simulink model "EPD_China_3_gen_without_limits"  (R2021b)
settings: Solver=VariableStepAuto  StartTime=0.0  StopTime=2  RelTol=1e-3
settings Model: Creator=vijay  LastModifiedBy=vijay

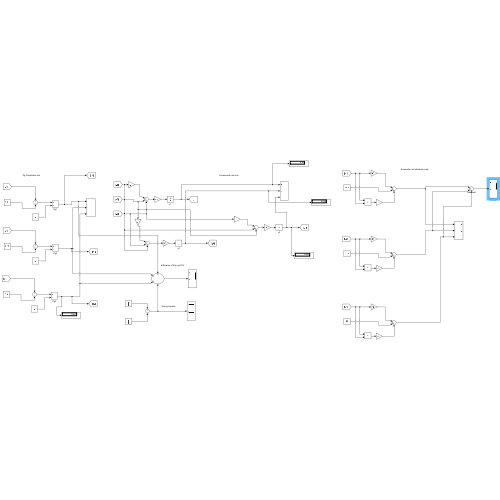
[thumbnail: Simulink's stored preview of the top-level diagram]
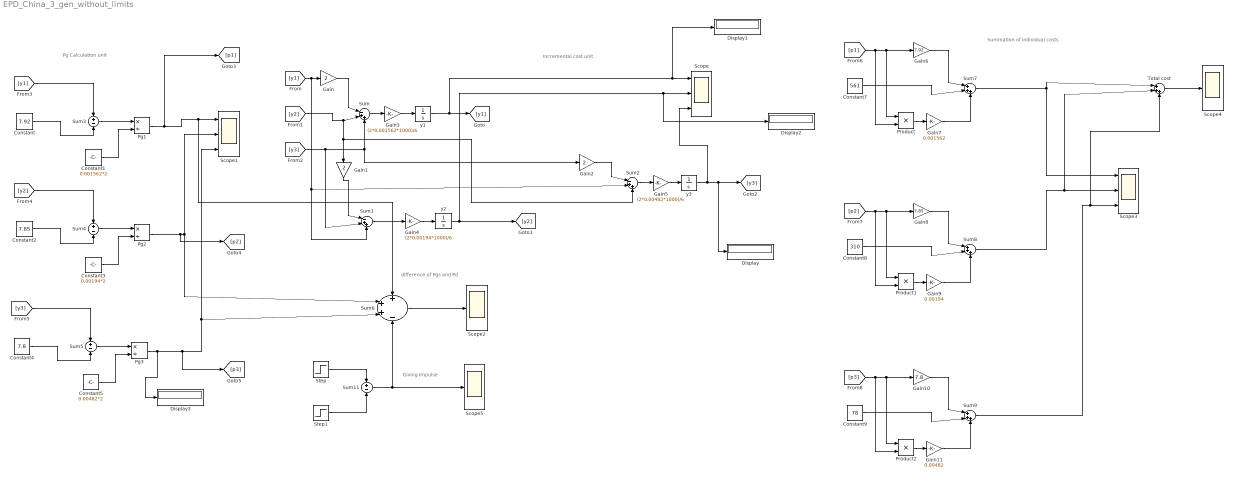
== system EPD_China_3_gen_without_limits ==
  note: Giving Impulse
  note: difference of Pgs and Pd
  note: Pg Calculation unit
  note: Summation of individual costs
  note: Incremental cost unit
  Constant : Constant  Value=7.92
  Constant1 : Constant  Value=0.001562*2
  Constant2 : Constant  Value=7.85
  Constant3 : Constant  Value=0.00194*2
  Constant4 : Constant  Value=7.8
  Constant5 : Constant  Value=0.00482*2
  Constant7 : Constant  Value=561
  Constant8 : Constant  Value=310
  Constant9 : Constant  Value=78
  Display{,1..3} (4 alike) : Display
  Gain : Gain  Gain=2
  Gain1 : Gain  Gain=2
  Gain10 : Gain  Gain=7.8
  Gain11 : Gain  Gain=0.00482
  Gain2 : Gain  Gain=2
  Gain3 : Gain  Gain=(2*0.001562*1000)/6
  Gain4 : Gain  Gain=(2*0.00194*1000)/6
  Gain5 : Gain  Gain=(2*0.00482*1000)/6
  Gain6 : Gain  Gain=7.92
  Gain7 : Gain  Gain=0.001562
  Gain8 : Gain  Gain=7.85
  Gain9 : Gain  Gain=0.00194
  Pg1 : Product  Inputs=*/
  Pg2 : Product  Inputs=*/
  Pg3 : Product  Inputs=*/
  Product : Product
  Product1 : Product
  Product2 : Product
  Scope : Scope  NumInputPorts=3
  Scope1 : Scope  NumInputPorts=3
  Scope2 : Scope
  Scope3 : Scope  NumInputPorts=3
  Scope4 : Scope
  Scope5 : Scope
  Step : Step  Time=0.025  After=650  SampleTime=0
  Step1 : Step  Time=0.05  After=650  SampleTime=0
  Sum : Sum  Inputs=|-++
  Sum1 : Sum  Inputs=|-++
  Sum{3..5,11} (4 alike) : Sum  Inputs=+-
  Sum2 : Sum  Inputs=|-++
  Sum6 : Sum  Inputs=+++-
  Sum7 : Sum  Inputs=|+++
  Sum8 : Sum  Inputs=|+++
  Sum9 : Sum  Inputs=|+++
  Total cost : Sum  Inputs=|+++
  y1 : Integrator  InitialCondition=8.8572
  y2 : Integrator  InitialCondition=8.82
  y3 : Integrator  InitialCondition=8.764
  wires:
  Sum/1 -> Gain3/1
  Sum1/1 -> Gain4/1
  Sum2/1 -> Gain5/1
  y1/1 -> Display1/1, Scope/1, [y1]
  y2/1 -> [y2], Display2/1, Scope/2
  y3/1 -> Scope/3, Display/1, [y3]
  [y1] -> Sum1/3, Sum2/2, Gain/1
  Gain/1 -> Sum/1
  [y2] -> Sum2/3, Gain1/1, Sum/2
  [y3] -> Sum1/2, Sum/3, Gain2/1
  Gain1/1 -> Sum1/1
  Gain2/1 -> Sum2/1
  [y1] -> Sum3/1
  Constant/1 -> Sum3/2
  Sum3/1 -> Pg1/1
  Constant1/1 -> Pg1/2
  [y2] -> Sum4/1
  Sum4/1 -> Pg2/1
  Constant2/1 -> Sum4/2
  Constant3/1 -> Pg2/2
  [y3] -> Sum5/1
  Sum5/1 -> Pg3/1
  Constant4/1 -> Sum5/2
  Constant5/1 -> Pg3/2
  Pg2/1 -> [p2], Scope1/2, Sum6/2
  Pg3/1 -> Display3/1, [p3], Scope1/3, Sum6/3
  Sum6/1 -> Scope2/1
  Gain3/1 -> y1/1
  Pg1/1 -> [p1], Sum6/1, Scope1/1
  Gain4/1 -> y2/1
  Gain5/1 -> y3/1
  Constant7/1 -> Sum7/2
  [p1] -> Product/2, Product/1, Gain6/1
  Gain6/1 -> Sum7/1
  Product/1 -> Gain7/1
  Gain7/1 -> Sum7/3
  Sum8/1 -> Total cost/2, Scope3/2
  Gain8/1 -> Sum8/1
  Gain9/1 -> Sum8/3
  Constant8/1 -> Sum8/2
  [p2] -> Product1/2, Product1/1, Gain8/1
  Product1/1 -> Gain9/1
  Sum9/1 -> Total cost/3, Scope3/3
  Gain10/1 -> Sum9/1
  Gain11/1 -> Sum9/3
  Constant9/1 -> Sum9/2
  [p3] -> Product2/2, Product2/1, Gain10/1
  Product2/1 -> Gain11/1
  Sum7/1 -> Scope3/1, Total cost/1
  Total cost/1 -> Scope4/1
  Step/1 -> Sum11/1
  Step1/1 -> Sum11/2
  Sum11/1 -> Scope5/1, Sum6/4
